simulink model "motordc"  (R2022b)
settings: Solver=VariableStepAuto  StartTime=0.0  StopTime=20  RelTol=1e-3
values from neighbouring files (symbols this model uses):
  A = [-R/L, -ke/L; kt/J, -c/J]    [sistdecontrolecomeficiencia.m]
  B = [1/L, 0; 0, -1/J]    [sistdecontrolecomeficiencia.m]
  C = [1, 0; 0, 1]    [sistdecontrolecomeficiencia.m]
  D = zeros(2, 2)    [sistdecontrolecomeficiencia.m]
settings Model: Creator=julin  LastModifiedBy=julin

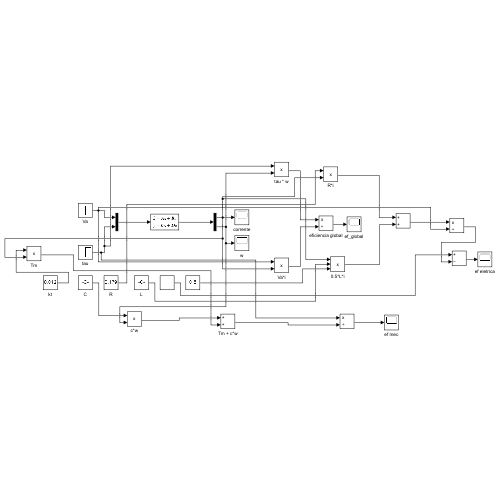
[thumbnail: Simulink's stored preview of the top-level diagram]
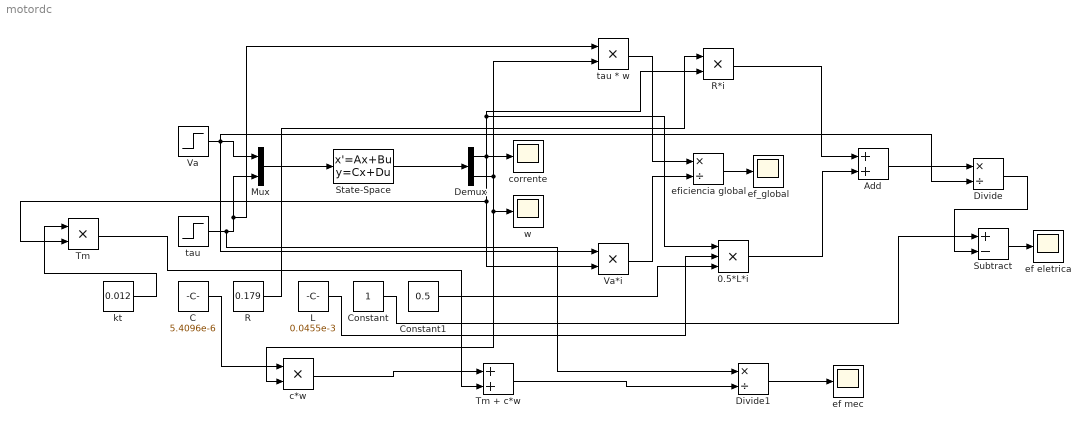
== system motordc ==
  0.5*L*i : Product  Inputs=3
  Add : Sum
  C : Constant  Value=5.4096e-6
  Constant : Constant
  Constant1 : Constant  Value=0.5
  Demux : Demux  Outputs=2
  Divide : Product  Inputs=*/
  Divide1 : Product  Inputs=*/
  L : Constant  Value=0.0455e-3
  Mux : Mux  Inputs=2
  R : Constant  Value=0.179
  R*i : Product
  State-Space : StateSpace  A=A  B=B  C=C  D=D  InitialCondition=0
  Subtract : Sum  Inputs=+-
  Tm : Product
  Tm + c*w : Sum
  Va : Step  Time=0  After=10  SampleTime=0
  Va*i : Product
  c*w : Product
  corrente : Scope
  ef eletrica : Scope
  ef mec : Scope
  ef_global : Scope
  eficiencia global : Product  Inputs=*/
  kt : Constant  Value=0.012
  tau : Step  Time=10  After=0.091  SampleTime=0
  tau * w : Product
  w : Scope
  wires:
  Mux/1 -> State-Space/1
  tau/1 -> Divide1/1, tau * w/1, Mux/2
  State-Space/1 -> Demux/1
  Demux/1 -> R*i/2, 0.5*L*i/1, Tm/2, Va*i/2, corrente/1
  Va/1 -> Divide/2, Va*i/1, Mux/1
  Demux/2 -> c*w/2, w/1, tau * w/2
  tau * w/1 -> eficiencia global/1
  Va*i/1 -> eficiencia global/2
  eficiencia global/1 -> ef_global/1
  L/1 -> 0.5*L*i/2
  R/1 -> R*i/1
  Constant1/1 -> 0.5*L*i/3
  R*i/1 -> Add/1
  0.5*L*i/1 -> Add/2
  Add/1 -> Divide/1
  Constant/1 -> Subtract/1
  Divide/1 -> Subtract/2
  Subtract/1 -> ef eletrica/1
  kt/1 -> Tm/1
  C/1 -> c*w/1
  c*w/1 -> Tm + c*w/1
  Tm/1 -> Tm + c*w/2
  Tm + c*w/1 -> Divide1/2
  Divide1/1 -> ef mec/1
